simulink model "expt"  (R2017a)
settings: Solver=VariableStepAuto  StartTime=0.0  StopTime=10.0  RelTol=1e-3
libraries: simulink x1
settings Model: Creator=jyotirmoy  LastModifiedBy=jyotirmoy

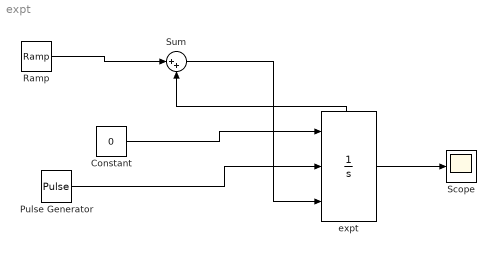
== system expt ==
  Constant : Constant  Value=0
  Pulse Generator : DiscretePulseGenerator  PulseType=Time based  Period=0.01  PulseWidth=5
  Ramp : simulink/Sources/Ramp  slope=1  start=0  X0=0
  Scope : Scope
  Sum : Sum  Inputs=|++
  expt : Integrator  ExternalReset=rising  InitialConditionSource=external  ShowStatePort=on
  wires:
  Constant/1 -> expt/1
  Pulse Generator/1 -> expt/2
  Ramp/1 -> Sum/1
  expt/State -> Sum/2
  Sum/1 -> expt/3
  expt/1 -> Scope/1
